simulink model "geometric_control__force_observer"  (R2021b)
settings: Solver=ode3  StartTime=0.0  StopTime=80  FixedStep=1e-2  RelTol=1e-3  EnableMultiTasking=on
libraries: sharedutil x7
settings Model: Creator=user
settings SolverCC: AlgebraicLoopSolver=TrustRegion  AutoInsertRateTranBlk=on
settings DataIOCC: LimitDataPoints=on  SaveFormat=Array  ReturnWorkspaceOutputs=off
settings OptimizationCC: ExpressionDepthLimit=2147483647  LifeSpan=inf
settings DebuggingCC: UnderspecifiedInitializationDetection=Classic  MergeDetectMultiDrivingBlocksExec=none  SolverPrmCheckMsg=warning  StateNameClashWarn=warning  SFUnexpectedBacktrackingDiag=warning  SFNoUnconditionalDefaultTransitionDiag=warning  SFExecutionAtInitializationDiag=none  SFMachineParentedDataDiag=warning  ArithmeticOperatorsInVariantConditions=warning
settings HardwareCC: ProdBitPerPointer=32  ProdBitPerSizeT=32  ProdBitPerPtrDiffT=32  ProdLargestAtomicFloat=None  ProdIntDivRoundTo=Undefined  ProdEndianess=Unspecified  ProdWordSize=32  ProdHWDeviceType=32-bit Generic
settings ModelReferenceCC: PropagateSignalLabelsOutOfModel=off
settings SFSimCC: SimUseLocalCustomCode=off  CustomCodeUndefinedFunction=UseInterfaceOnly
settings RTWCC: RTWUseLocalCustomCode=off
settings CodeAppCC: StateflowObjectComments=on
settings GRTTargetCC: TargetLangStandard=C89/C90 (ANSI)
settings ConfigComp: CovMetricSettings=dw  CovSaveCumulativeToWorkspaceVar=on  CovSaveSingleToWorkspaceVar=on  CovExternalEMLEnable=off

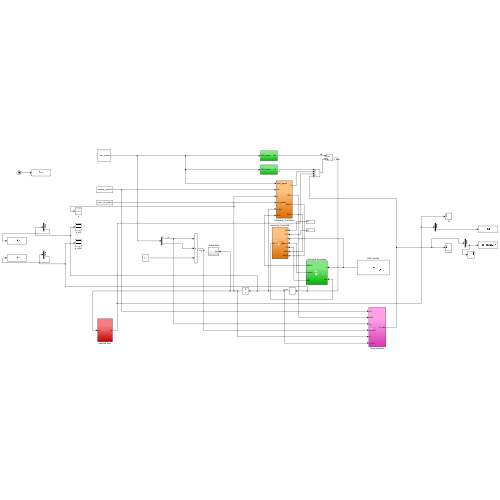
[thumbnail: Simulink's stored preview of the top-level diagram]
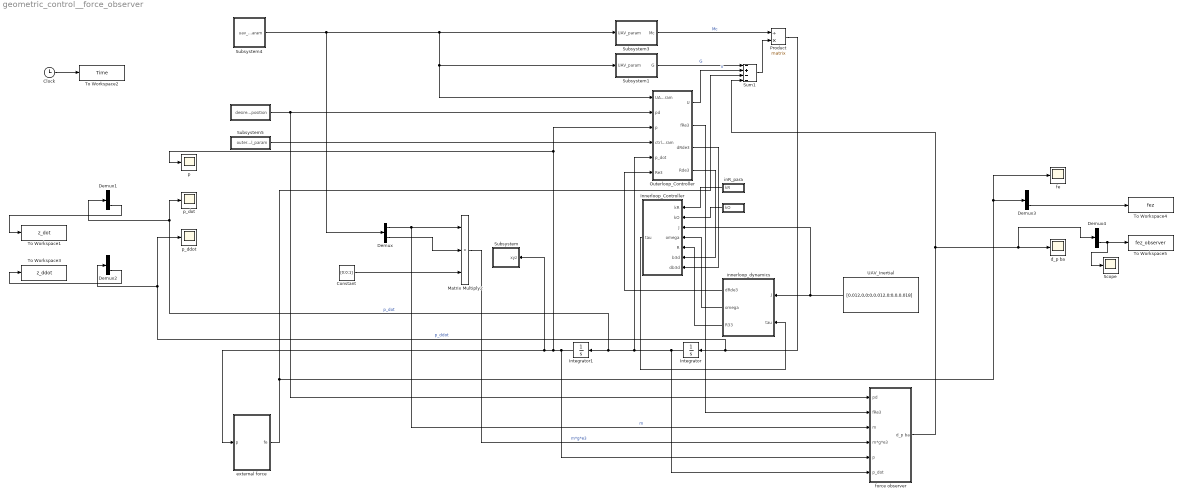
== system geometric_control__force_observer ==
  " " : Subsystem  mask{xd=3, yd=6, zd=10}
  "  " : Subsystem  mask{kO=diag([0.6,0.6,1])}
  "  Subsystem" : Subsystem
  Clock : Clock
  Constant : Constant  Value=[0;0;1]
  Demux : Demux  Outputs=2
  Demux{1..4} (4 alike) : Demux  Outputs=3
  Innerloop_Controller : Subsystem
  Integrator : Integrator  InitialCondition=[0;0;0]
  Integrator1 : Integrator  InitialCondition=[0;0;0]
  Matrix Multiply2 : Product  Inputs=3
  Outerloop_Controller : Subsystem
  Product : Product  Inputs=/*  Multiplication=Matrix(*)  RndMeth=Zero
  Scope : Scope
  Subsystem1 : Subsystem
  Subsystem3 : Subsystem
  Subsystem4 : Subsystem  mask{M=1.4, g=9.8}
  Subsystem5 : Subsystem  mask{kp1=0.1, kd1=1, kp2=0.5, kd2=3, kp3=0.05, kd3=0.5}
  Sum1 : Sum  Inputs=-+--
  To Workspace1 : ToWorkspace  VariableName=z_dot  SaveFormat=Structure With Time  SampleTime=-1
  To Workspace2 : ToWorkspace  VariableName=Time  SaveFormat=Timeseries  SampleTime=-1
  To Workspace3 : ToWorkspace  VariableName=z_ddot  SaveFormat=Structure With Time  SampleTime=-1
  To Workspace4 : ToWorkspace  VariableName=fez  SaveFormat=Structure With Time  SampleTime=-1
  To Workspace5 : ToWorkspace  VariableName=fez_observer  SaveFormat=Structure With Time  SampleTime=-1
  UAV_Inertial : Constant  Value=[0.012,0,0;0,0.012,0;0,0,0.018]
  d_p ba : Scope
  external force : Subsystem
  fe : Scope
  force observer : Subsystem
  inR_para : Subsystem  mask{kR=diag([5,5,4.7])}
  innerloop_dynamics : Subsystem
  p : Scope
  p_ddot : Scope
  p_dot : Scope
  wires:
  Subsystem3/1("Mc ") -> Product/1  "Mc"
  Product/1 -> p_ddot/1, Demux2/1, Integrator/1  "p_ddot"
  Subsystem4/1(uav_param) -> Outerloop_Controller/1(UAV_param), Subsystem1/1(UAV_param), Subsystem3/1(UAV_param), Demux/1
  Outerloop_Controller/1(U) -> Sum1/2  "u"
  Outerloop_Controller/3(dRde3) -> Innerloop_Controller/7(db3d)
  Outerloop_Controller/4(Rde3) -> Innerloop_Controller/6(b3d)
  UAV_Inertial/1 -> Innerloop_Controller/3(J), innerloop_dynamics/1(J)
  innerloop_dynamics/2(omega) -> Innerloop_Controller/4(omega)
  innerloop_dynamics/3(R33) -> Innerloop_Controller/5(R)
  Subsystem1/1("G ") -> Sum1/1  "G"
  Sum1/1 -> Product/2
  Innerloop_Controller/1(tau) -> innerloop_dynamics/2(tau)
  innerloop_dynamics/1(dRde3) -> Outerloop_Controller/6(Re3)
  Subsystem5/1(outer_ctrl_param) -> Outerloop_Controller/4(ctrl_param)
  Integrator/1 -> Demux1/1, p_dot/1, Integrator1/1, Outerloop_Controller/5(p_dot), force observer/6(p_dot)  "p_dot"
  "  "/1(kO) -> Innerloop_Controller/2(kO)
  inR_para/1(kR) -> Innerloop_Controller/1(kR)
  Demux/1 -> force observer/3(m), Matrix Multiply2/1  "m"
  Demux/2 -> Matrix Multiply2/2
  Constant/1 -> Matrix Multiply2/3
  " "/1(desired_position) -> Outerloop_Controller/2(pd), force observer/1(pd)
  Integrator1/1 -> external force/1(p), "  Subsystem"/1(xyz), Outerloop_Controller/3(p), p/1, force observer/5(p)
  external force/1(fe) -> Demux3/1, fe/1, Sum1/3
  Outerloop_Controller/2(fRe3) -> force observer/2(fRe3)
  Matrix Multiply2/1 -> force observer/4(m*g*e3)  "m*g*e3"
  force observer/1(d_p ba) -> Sum1/4, Demux4/1, d_p ba/1
  Clock/1 -> To Workspace2/1
  Demux1/3 -> To Workspace1/1
  Demux2/3 -> To Workspace3/1
  Demux3/3 -> To Workspace4/1
  Demux4/3 -> Scope/1, To Workspace5/1

== system geometric_control__force_observer/  ==
  Constant : Constant  Value=xd
  Constant1 : Constant  Value=zd
  Constant2 : Constant  Value=yd
  Mux : Mux  Inputs=3
  desired_position : Outport
  wires:
  Constant/1 -> Mux/1
  Constant2/1 -> Mux/2
  Mux/1 -> desired_position/1
  Constant1/1 -> Mux/3

== system geometric_control__force_observer/   ==
  Constant1 : Constant  Value=kO
  kO : Outport
  wires:
  Constant1/1 -> kO/1

== system geometric_control__force_observer/  Subsystem ==
  xyz : Inport
  Demux : Demux  Outputs=3
  To Workspace : ToWorkspace  VariableName=x  SaveFormat=Structure With Time  SampleTime=-1
      settings: Save2DSignal=2-D array (concatenate along first dimension)
  To Workspace2 : ToWorkspace  VariableName=y  SaveFormat=Structure With Time  SampleTime=-1
      settings: Save2DSignal=2-D array (concatenate along first dimension)
  To Workspace3 : ToWorkspace  VariableName=z  SaveFormat=Structure With Time  SampleTime=-1
      settings: Save2DSignal=2-D array (concatenate along first dimension)
  wires:
  Demux/3 -> To Workspace3/1
  Demux/1 -> To Workspace/1
  Demux/2 -> To Workspace2/1
  xyz/1 -> Demux/1

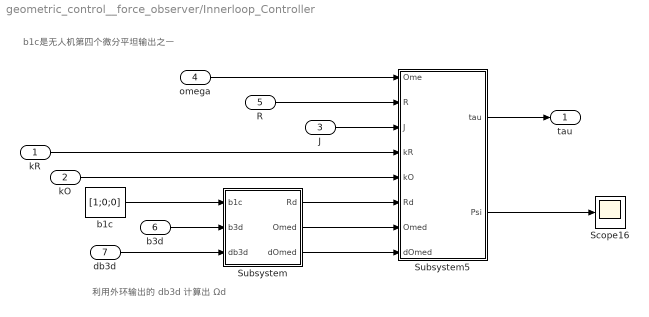
== system geometric_control__force_observer/Innerloop_Controller ==
  note: 利用外环输出的 db3d 计算出 Ωd
  note: b1c是无人机第四个微分平坦输出之一
  kR : Inport
  kO : Inport  Port=2
  J : Inport  Port=3
  omega : Inport  Port=4
  R : Inport  Port=5
  b3d : Inport  Port=6
  db3d : Inport  Port=7
  Scope16 : Scope
  Subsystem : Subsystem
  Subsystem5 : Subsystem
  b1c : Constant  Value=[1;0;0]
  tau : Outport
  wires:
  b1c/1 -> Subsystem/1(b1c)
  Subsystem5/2(Psi) -> Scope16/1
  db3d/1 -> Subsystem/3(db3d)
  kR/1 -> Subsystem5/4(kR)
  Subsystem/2(Omed) -> Subsystem5/7(Omed)
  Subsystem/1(Rd) -> Subsystem5/6(Rd)
  b3d/1 -> Subsystem/2(b3d)
  Subsystem/3(dOmed) -> Subsystem5/8(dOmed)
  kO/1 -> Subsystem5/5(kO)
  omega/1 -> Subsystem5/1(Ome)
  R/1 -> Subsystem5/2(R)
  J/1 -> Subsystem5/3(J)
  Subsystem5/1(tau) -> tau/1

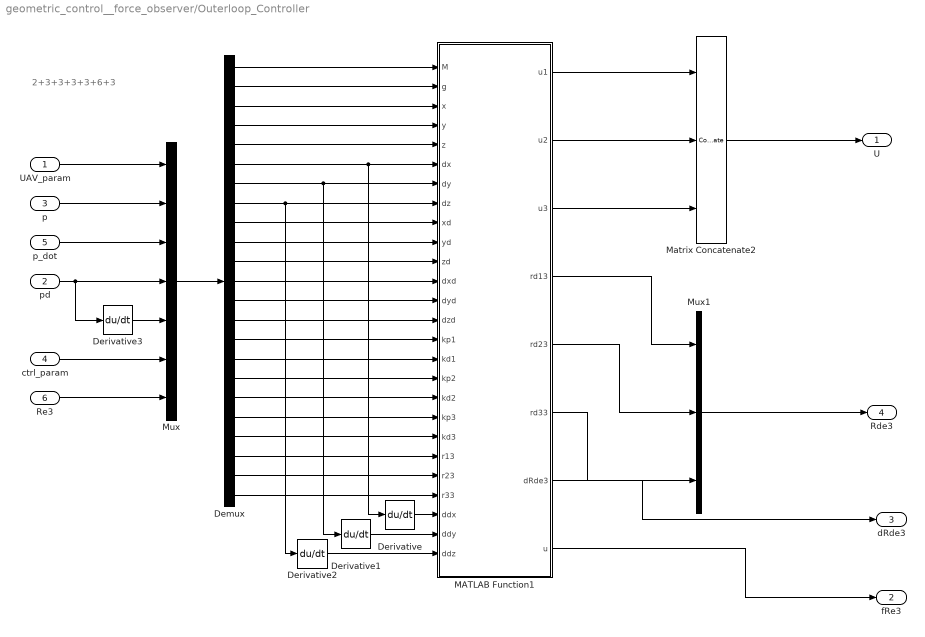
== system geometric_control__force_observer/Outerloop_Controller ==
  note: 2+3+3+3+3+6+3
  UAV_param : Inport
  pd : Inport  Port=2
  p : Inport  Port=3
  ctrl_param : Inport  Port=4
  p_dot : Inport  Port=5
  Re3 : Inport  Port=6
  Demux : Demux  Outputs=23
  Derivative{,1..3} (4 alike) : Derivative
  MATLAB Function1 : MATLAB Function  TreatAsAtomicUnit=on
  Matrix Concatenate2 : Concatenate  NumInputs=3  Mode=Multidimensional array
  Mux : Mux  Inputs=7
  Mux1 : Mux  Inputs=3
  U : Outport
  fRe3 : Outport  Port=2
  dRde3 : Outport  Port=3
  Rde3 : Outport  Port=4
  wires:
  Matrix Concatenate2/1 -> U/1
  UAV_param/1 -> Mux/1
  Mux/1 -> Demux/1
  Mux1/1 -> Rde3/1
  p_dot/1 -> Mux/3
  ctrl_param/1 -> Mux/6
  Re3/1 -> Mux/7
  p/1 -> Mux/2
  Demux/1 -> MATLAB Function1/1(M)
  Demux/2 -> MATLAB Function1/2(g)
  Demux/3 -> MATLAB Function1/3(x)
  Demux/4 -> MATLAB Function1/4(y)
  Demux/5 -> MATLAB Function1/5(z)
  Demux/6 -> Derivative/1, MATLAB Function1/6(dx)
  Demux/7 -> MATLAB Function1/7(dy), Derivative1/1
  Demux/8 -> Derivative2/1, MATLAB Function1/8(dz)
  Demux/9 -> MATLAB Function1/9(xd)
  Demux/10 -> MATLAB Function1/10(yd)
  Demux/11 -> MATLAB Function1/11(zd)
  Demux/12 -> MATLAB Function1/12(dxd)
  Demux/13 -> MATLAB Function1/13(dyd)
  Demux/14 -> MATLAB Function1/14(dzd)
  Demux/15 -> MATLAB Function1/15(kp1)
  Demux/16 -> MATLAB Function1/16(kd1)
  Demux/17 -> MATLAB Function1/17(kp2)
  Demux/18 -> MATLAB Function1/18(kd2)
  Demux/19 -> MATLAB Function1/19(kp3)
  Demux/20 -> MATLAB Function1/20(kd3)
  Demux/21 -> MATLAB Function1/21(r13)
  Demux/22 -> MATLAB Function1/22(r23)
  Demux/23 -> MATLAB Function1/23(r33)
  MATLAB Function1/1(u1) -> Matrix Concatenate2/1
  MATLAB Function1/2(u2) -> Matrix Concatenate2/2
  MATLAB Function1/3(u3) -> Matrix Concatenate2/3
  MATLAB Function1/4(rd13) -> Mux1/1
  MATLAB Function1/5(rd23) -> Mux1/2
  MATLAB Function1/6(rd33) -> Mux1/3
  MATLAB Function1/7(dRde3) -> dRde3/1
  Derivative/1 -> MATLAB Function1/24(ddx)
  Derivative1/1 -> MATLAB Function1/25(ddy)
  Derivative2/1 -> MATLAB Function1/26(ddz)
  pd/1 -> Derivative3/1, Mux/4
  Derivative3/1 -> Mux/5
  MATLAB Function1/8(u) -> fRe3/1

== system geometric_control__force_observer/Subsystem1 ==
  UAV_param : Inport
  G1 : Fcn  Expr=0*u(1)
  G2 : Fcn  Expr=0*u(1)
  G3 : Fcn  Expr=u(1)*u(2)
  Matrix Concatenate2 : Concatenate  NumInputs=3  Mode=Multidimensional array
  "G " : Outport
  wires:
  UAV_param/1 -> G1/1, G2/1, G3/1
  Matrix Concatenate2/1 -> "G "/1
  G3/1 -> Matrix Concatenate2/3
  G2/1 -> Matrix Concatenate2/2
  G1/1 -> Matrix Concatenate2/1

== system geometric_control__force_observer/Subsystem3 ==
  UAV_param : Inport
  Matrix Concatenate2 : Concatenate  NumInputs=3  Mode=Multidimensional array  ConcatenateDimension=2
  Subsystem : Subsystem
  Subsystem1 : Subsystem
  Subsystem2 : Subsystem
  "Mc " : Outport
  wires:
  UAV_param/1 -> Subsystem/1((S,p)), Subsystem1/1((S,p)), Subsystem2/1((S,p))
  Matrix Concatenate2/1 -> "Mc "/1
  Subsystem2/1(Mc3) -> Matrix Concatenate2/3
  Subsystem1/1(Mc2) -> Matrix Concatenate2/2
  Subsystem/1(Mc1) -> Matrix Concatenate2/1

== system geometric_control__force_observer/Subsystem4 ==
  Constant : Constant  Value=M
  Constant2 : Constant  Value=g
  Mux : Mux  Inputs=2
  uav_param : Outport
  wires:
  Constant/1 -> Mux/1
  Constant2/1 -> Mux/2
  Mux/1 -> uav_param/1

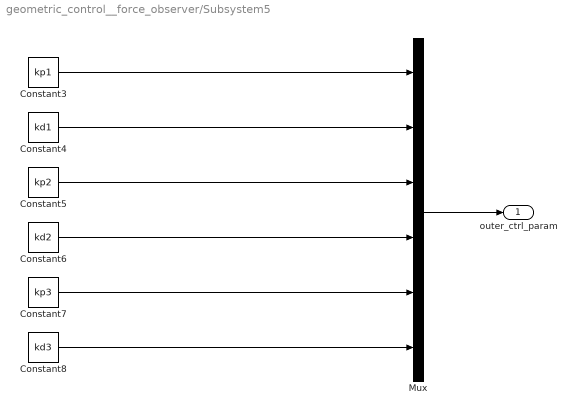
== system geometric_control__force_observer/Subsystem5 ==
  Constant3 : Constant  Value=kp1
  Constant4 : Constant  Value=kd1
  Constant5 : Constant  Value=kp2
  Constant6 : Constant  Value=kd2
  Constant7 : Constant  Value=kp3
  Constant8 : Constant  Value=kd3
  Mux : Mux  Inputs=6
  outer_ctrl_param : Outport
  wires:
  Mux/1 -> outer_ctrl_param/1
  Constant3/1 -> Mux/1
  Constant4/1 -> Mux/2
  Constant5/1 -> Mux/3
  Constant6/1 -> Mux/4
  Constant7/1 -> Mux/5
  Constant8/1 -> Mux/6

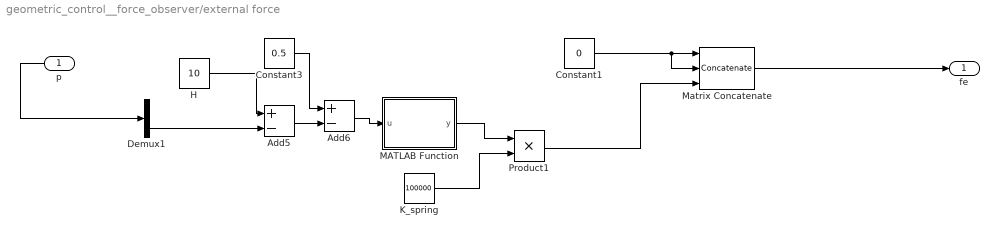
== system geometric_control__force_observer/external force ==
  p : Inport
  Add5 : Sum  Inputs=+-
  Add6 : Sum  Inputs=+-
  Constant1 : Constant  Value=0
  Constant3 : Constant  Value=0.5
  Demux1 : Demux  Outputs=3
  H : Constant  Value=10
  K_spring : Constant  Value=100000
  MATLAB Function : MATLAB Function  TreatAsAtomicUnit=on
  Matrix Concatenate : Concatenate  NumInputs=3  Mode=Multidimensional array
  Product1 : Product
  fe : Outport
  wires:
  H/1 -> Add5/1
  Product1/1 -> Matrix Concatenate/3
  Add5/1 -> Add6/2
  Matrix Concatenate/1 -> fe/1
  MATLAB Function/1(y) -> Product1/1
  K_spring/1 -> Product1/2
  Add6/1 -> MATLAB Function/1(u)
  p/1 -> Demux1/1
  Demux1/3 -> Add5/2
  Constant3/1 -> Add6/1
  Constant1/1 -> Matrix Concatenate/2, Matrix Concatenate/1

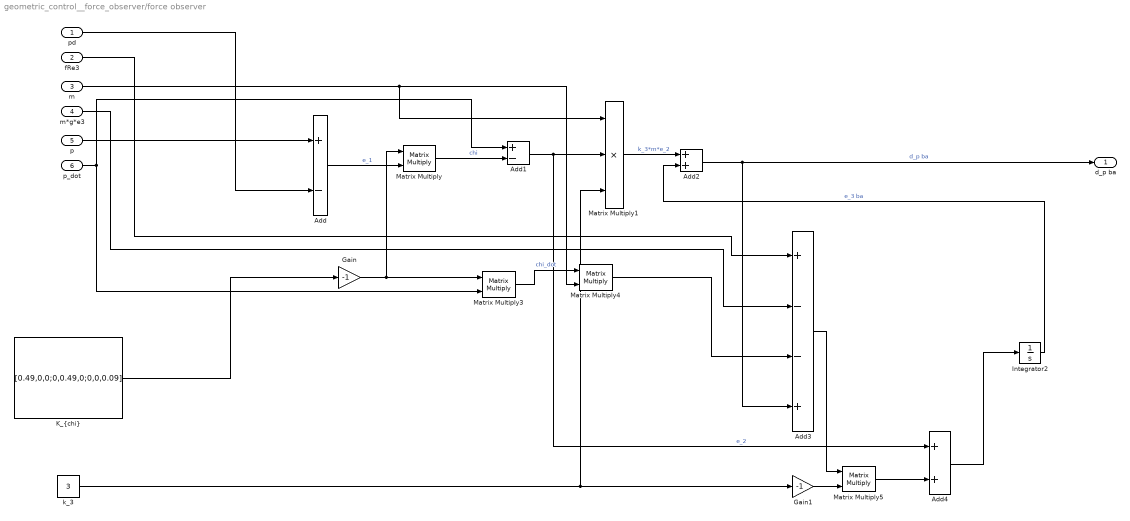
== system geometric_control__force_observer/force observer ==
  pd : Inport
  fRe3 : Inport  Port=2
  m : Inport  Port=3
  m*g*e3 : Inport  Port=4
  p : Inport  Port=5
  p_dot : Inport  Port=6
  Add : Sum  Inputs=+-
  Add1 : Sum  Inputs=+-
  Add2 : Sum
  Add3 : Sum  Inputs=+--+
  Add4 : Sum
  Gain : Gain  Gain=-1
  Gain1 : Gain  Gain=-1
  Integrator2 : Integrator
  "K_{chi}" : Constant  Value=[0.49,0,0;0,0.49,0;0,0,0.09]
  Matrix Multiply{,3..5} (4 alike) : Product  Multiplication=Matrix(*)
  Matrix Multiply1 : Product  Inputs=3
  k_3 : Constant  Value=3
  d_p ba : Outport
  wires:
  Add2/1 -> d_p ba/1, Add3/4  "d_p ba"
  Gain/1 -> Matrix Multiply/1, Matrix Multiply3/1
  Add4/1 -> Integrator2/1
  p_dot/1 -> Add1/1, Matrix Multiply3/2
  p/1 -> Add/1
  Matrix Multiply4/1 -> Add3/3
  Add1/1 -> Add4/1, Matrix Multiply1/2  "e_2"
  k_3/1 -> Matrix Multiply1/3, Gain1/1
  Add/1 -> Matrix Multiply/2  "e_1"
  Matrix Multiply1/1 -> Add2/1  "k_3*m*e_2"
  fRe3/1 -> Add3/1
  Integrator2/1 -> Add2/2  "e_3 ba"
  m/1 -> Matrix Multiply1/1, Matrix Multiply4/2
  Matrix Multiply3/1 -> Matrix Multiply4/1  "chi_dot"
  Matrix Multiply/1 -> Add1/2  "chi"
  "K_{chi}"/1 -> Gain/1
  Matrix Multiply5/1 -> Add4/2
  Add3/1 -> Matrix Multiply5/1
  Gain1/1 -> Matrix Multiply5/2
  m*g*e3/1 -> Add3/2
  pd/1 -> Add/2

== system geometric_control__force_observer/inR_para ==
  Constant : Constant  Value=kR
  kR : Outport
  wires:
  Constant/1 -> kR/1

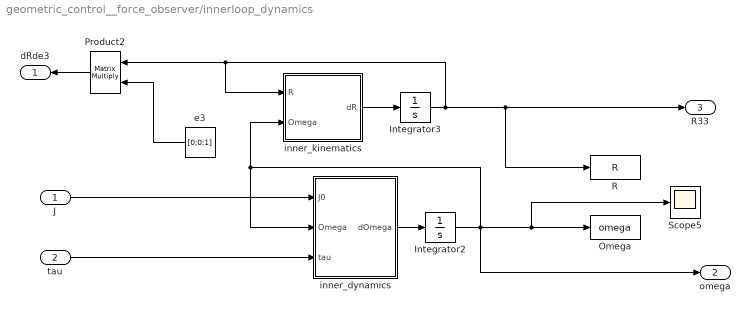
== system geometric_control__force_observer/innerloop_dynamics ==
  J : Inport
  tau : Inport  Port=2
  Integrator2 : Integrator  InitialCondition=[0;0;0]
  Integrator3 : Integrator  InitialCondition=[1,0,0;0,1,0;0,0,1]
  Omega : ToWorkspace  VariableName=omega  SampleTime=-1
  Product2 : Product  Multiplication=Matrix(*)  RndMeth=Zero
  R : ToWorkspace  VariableName=R  SampleTime=-1
  Scope5 : Scope
  e3 : Constant  Value=[0;0;1]
  inner_dynamics : Subsystem
  inner_kinematics : Subsystem
  dRde3 : Outport
  omega : Outport  Port=2
  R33 : Outport  Port=3
  wires:
  inner_kinematics/1(dR) -> Integrator3/1
  Product2/1 -> dRde3/1
  Integrator3/1 -> inner_kinematics/1(R), Product2/1, R/1, R33/1
  Integrator2/1 -> Omega/1, Scope5/1, inner_dynamics/2(Omega), inner_kinematics/2(Omega), omega/1
  e3/1 -> Product2/2
  inner_dynamics/1(dOmega) -> Integrator2/1
  J/1 -> inner_dynamics/1(J0)
  tau/1 -> inner_dynamics/3(tau)

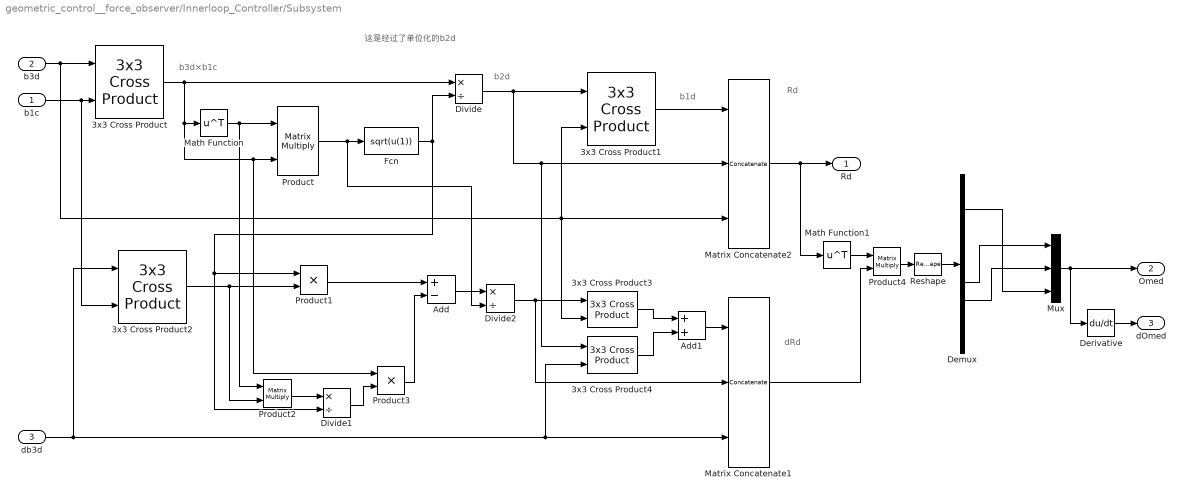
== system geometric_control__force_observer/Innerloop_Controller/Subsystem ==
  note: 这是经过了单位化的b2d
  note: b3d×b1c
  note: dRd
  note: Rd
  note: b1d
  note: b2d
  b1c : Inport
  b3d : Inport  Port=2
  db3d : Inport  Port=3
  3x3 Cross Product{,1..4} (5 alike) : sharedutil/3x3 Cross Product  aMode=aMode
      settings: SourceProductBaseCode=AE,PW,DR,MT,UV,VE
  Add : Sum  Inputs=+-
  Add1 : Sum
  Demux : Demux  Outputs=9
  Derivative : Derivative
  Divide : Product  Inputs=*/
  Divide1 : Product  Inputs=*/
  Divide2 : Product  Inputs=*/
  Fcn : Fcn  Expr=sqrt(u(1))
  Math Function : Math  Operator=transpose  SignedPower=on  SaturateOnIntegerOverflow=on
  Math Function1 : Math  Operator=transpose  SignedPower=on  SaturateOnIntegerOverflow=on
  Matrix Concatenate1 : Concatenate  NumInputs=3  Mode=Multidimensional array  ConcatenateDimension=2
  Matrix Concatenate2 : Concatenate  NumInputs=3  Mode=Multidimensional array  ConcatenateDimension=2
  Mux : Mux  Inputs=3
  Product : Product  Multiplication=Matrix(*)  RndMeth=Zero
  Product1 : Product  RndMeth=Zero
  Product2 : Product  Multiplication=Matrix(*)  RndMeth=Zero
  Product3 : Product  RndMeth=Zero
  Product4 : Product  Multiplication=Matrix(*)  RndMeth=Zero
  Reshape : Reshape
  Rd : Outport
  Omed : Outport  Port=2
  dOmed : Outport  Port=3
  wires:
  b3d/1 -> 3x3 Cross Product1/2, Matrix Concatenate2/3, 3x3 Cross Product3/2, 3x3 Cross Product/1
  b1c/1 -> 3x3 Cross Product2/2, 3x3 Cross Product/2
  3x3 Cross Product/1 -> Product3/1, Product/2, Math Function/1, Divide/1
  Math Function/1 -> Product/1, Product2/1
  Product/1 -> Divide2/2, Fcn/1
  Fcn/1 -> Divide1/2, Product1/1, Divide/2
  3x3 Cross Product1/1 -> Matrix Concatenate2/1
  db3d/1 -> 3x3 Cross Product2/1, 3x3 Cross Product4/2, Matrix Concatenate1/3
  3x3 Cross Product2/1 -> Product2/2, Product1/2
  Product1/1 -> Add/1
  Product2/1 -> Divide1/1
  Divide1/1 -> Product3/2
  Product3/1 -> Add/2
  Add/1 -> Divide2/1
  Divide2/1 -> 3x3 Cross Product3/1, Matrix Concatenate1/2
  3x3 Cross Product3/1 -> Add1/1
  3x3 Cross Product4/1 -> Add1/2
  Add1/1 -> Matrix Concatenate1/1
  Divide/1 -> 3x3 Cross Product4/1, Matrix Concatenate2/2, 3x3 Cross Product1/1
  Matrix Concatenate2/1 -> Math Function1/1, Rd/1
  Matrix Concatenate1/1 -> Product4/2
  Math Function1/1 -> Product4/1
  Demux/2 -> Mux/3
  Demux/6 -> Mux/1
  Demux/7 -> Mux/2
  Mux/1 -> Derivative/1, Omed/1
  Derivative/1 -> dOmed/1
  Reshape/1 -> Demux/1
  Product4/1 -> Reshape/1

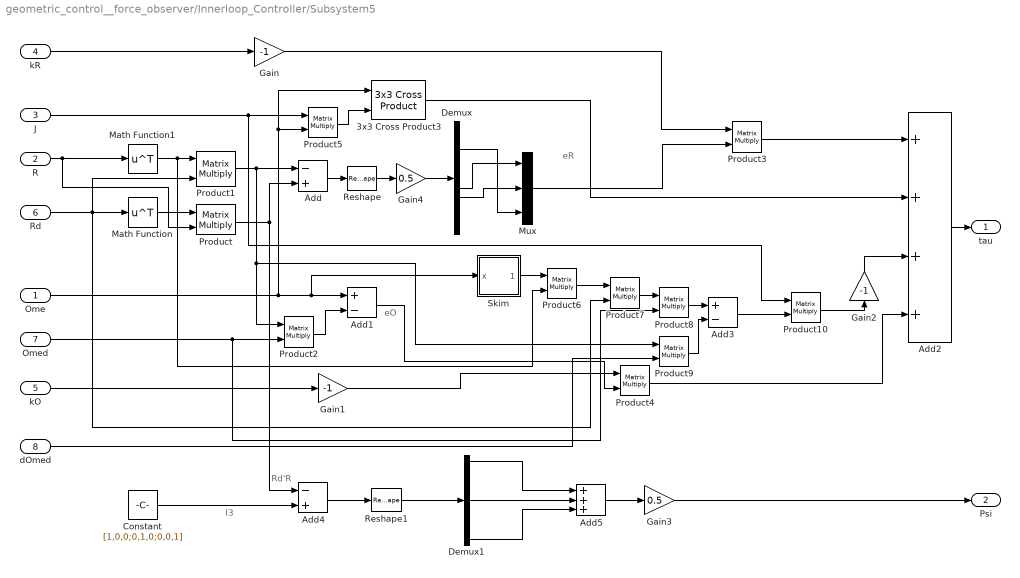
== system geometric_control__force_observer/Innerloop_Controller/Subsystem5 ==
  note: Rd'R
  note: I3
  note: eO
  note: eR
  Ome : Inport
  R : Inport  Port=2
  J : Inport  Port=3
  kR : Inport  Port=4
  kO : Inport  Port=5
  Rd : Inport  Port=6
  Omed : Inport  Port=7
  dOmed : Inport  Port=8
  3x3 Cross Product3 : sharedutil/3x3 Cross Product  aMode=aMode
      settings: SourceProductBaseCode=AE,PW,DR,MT,UV,VE
  Add : Sum  Inputs=-+
  Add1 : Sum  Inputs=+-
  Add2 : Sum  Inputs=++++
  Add3 : Sum  Inputs=+-
  Add4 : Sum  Inputs=-+
  Add5 : Sum  Inputs=+++
  Constant : Constant  Value=[1,0,0;0,1,0;0,0,1]
  Demux : Demux  Outputs=9
  Demux1 : Demux  Outputs=9
  Gain : Gain  Gain=-1
  Gain1 : Gain  Gain=-1
  Gain2 : Gain  Gain=-1
  Gain3 : Gain  Gain=0.5
  Gain4 : Gain  Gain=0.5
  Math Function : Math  Operator=transpose  SignedPower=on  SaturateOnIntegerOverflow=on
  Math Function1 : Math  Operator=transpose  SignedPower=on  SaturateOnIntegerOverflow=on
  Mux : Mux  Inputs=3
  Product{,1..10} (11 alike) : Product  Multiplication=Matrix(*)  RndMeth=Zero
  Reshape : Reshape
  Reshape1 : Reshape
  Skim : Subsystem
  tau : Outport
  Psi : Outport  Port=2
  wires:
  R/1 -> Product/2, Math Function1/1
  Rd/1 -> Product1/2, Math Function/1, Product7/2
  Math Function1/1 -> Product6/2, Product1/1
  Product1/1 -> Product9/1, Product2/1, Add/1
  Product/1 -> Add/2, Add4/1
  Add/1 -> Reshape/1
  Reshape/1 -> Gain4/1
  Demux/2 -> Mux/3
  Demux/6 -> Mux/1
  Demux/7 -> Mux/2
  Omed/1 -> Product8/2, Product2/2
  Ome/1 -> 3x3 Cross Product3/1, Product5/2, Skim/1(x), Add1/1
  Product2/1 -> Add1/2
  kR/1 -> Gain/1
  Mux/1 -> Product3/2
  Gain/1 -> Product3/1
  kO/1 -> Gain1/1
  Gain1/1 -> Product4/1
  Add1/1 -> Product4/2
  Add2/1 -> tau/1
  J/1 -> Product10/1, Product5/1
  Product5/1 -> 3x3 Cross Product3/2
  3x3 Cross Product3/1 -> Add2/2
  Product3/1 -> Add2/1
  Product4/1 -> Add2/4
  Skim/1(sk(x)) -> Product6/1
  Product6/1 -> Product7/1
  Product7/1 -> Product8/1
  Product8/1 -> Add3/1
  dOmed/1 -> Product9/2
  Product9/1 -> Add3/2
  Add3/1 -> Product10/2
  Product10/1 -> Gain2/1
  Gain2/1 -> Add2/3
  Math Function/1 -> Product/1
  Constant/1 -> Add4/2
  Reshape1/1 -> Demux1/1
  Add4/1 -> Reshape1/1
  Demux1/1 -> Add5/1
  Demux1/5 -> Add5/2
  Demux1/9 -> Add5/3
  Add5/1 -> Gain3/1
  Gain3/1 -> Psi/1
  Gain4/1 -> Demux/1

== system geometric_control__force_observer/Subsystem3/Subsystem ==
  (S,p) : Inport
  Matrix Concatenate2 : Concatenate  NumInputs=3  Mode=Multidimensional array
  Mc11 : Fcn  Expr=u(1)
  Mc21 : Fcn  Expr=0*u(1)
  Mc31 : Fcn  Expr=0*u(1)
  Mc1 : Outport
  wires:
  (S,p)/1 -> Mc11/1, Mc31/1, Mc21/1
  Mc11/1 -> Matrix Concatenate2/1
  Mc21/1 -> Matrix Concatenate2/2
  Mc31/1 -> Matrix Concatenate2/3
  Matrix Concatenate2/1 -> Mc1/1

== system geometric_control__force_observer/Subsystem3/Subsystem1 ==
  (S,p) : Inport
  Matrix Concatenate2 : Concatenate  NumInputs=3  Mode=Multidimensional array
  Mc12 : Fcn  Expr=0*u(1)
  Mc22 : Fcn  Expr=u(1)
  Mc32 : Fcn  Expr=0*u(1)
  Mc2 : Outport
  wires:
  (S,p)/1 -> Mc22/1, Mc32/1, Mc12/1
  Mc12/1 -> Matrix Concatenate2/1
  Mc22/1 -> Matrix Concatenate2/2
  Mc32/1 -> Matrix Concatenate2/3
  Matrix Concatenate2/1 -> Mc2/1

== system geometric_control__force_observer/Subsystem3/Subsystem2 ==
  (S,p) : Inport
  Matrix Concatenate2 : Concatenate  NumInputs=3  Mode=Multidimensional array
  Mc13 : Fcn  Expr=0*u(1)
  Mc23 : Fcn  Expr=0*u(1)
  Mc33 : Fcn  Expr=u(1)
  Mc3 : Outport
  wires:
  (S,p)/1 -> Mc23/1, Mc33/1, Mc13/1
  Mc13/1 -> Matrix Concatenate2/1
  Mc23/1 -> Matrix Concatenate2/2
  Mc33/1 -> Matrix Concatenate2/3
  Matrix Concatenate2/1 -> Mc3/1

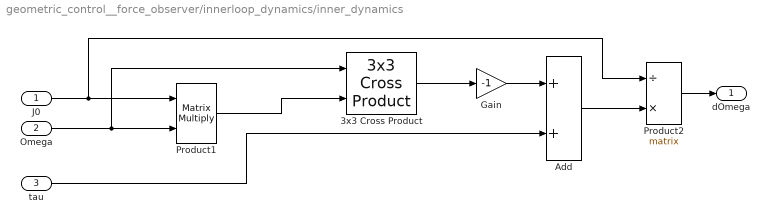
== system geometric_control__force_observer/innerloop_dynamics/inner_dynamics ==
  J0 : Inport
  Omega : Inport  Port=2
  tau : Inport  Port=3
  3x3 Cross Product : sharedutil/3x3 Cross Product  aMode=aMode
      settings: SourceProductBaseCode=AE,PW,DR,MT,UV,VE
  Add : Sum
  Gain : Gain  Gain=-1
  Product1 : Product  Multiplication=Matrix(*)  RndMeth=Zero
  Product2 : Product  Inputs=/*  Multiplication=Matrix(*)  RndMeth=Zero
  dOmega : Outport
  wires:
  J0/1 -> Product1/1, Product2/1
  Omega/1 -> 3x3 Cross Product/1, Product1/2
  Product1/1 -> 3x3 Cross Product/2
  3x3 Cross Product/1 -> Gain/1
  Gain/1 -> Add/1
  tau/1 -> Add/2
  Add/1 -> Product2/2
  Product2/1 -> dOmega/1

== system geometric_control__force_observer/innerloop_dynamics/inner_kinematics ==
  R : Inport
  Omega : Inport  Port=2
  Product1 : Product  Multiplication=Matrix(*)  RndMeth=Zero
  Skew : Subsystem
  dR : Outport
  wires:
  Omega/1 -> Skew/1(Omega)
  R/1 -> Product1/1
  Skew/1(OmegaX) -> Product1/2
  Product1/1 -> dR/1

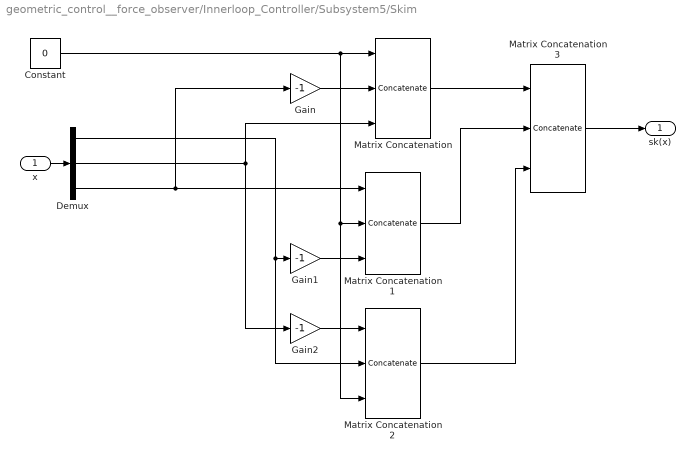
== system geometric_control__force_observer/Innerloop_Controller/Subsystem5/Skim ==
  x : Inport
  Constant : Constant  Value=0
  Demux : Demux  Outputs=3
  Gain : Gain  Gain=-1
  Gain1 : Gain  Gain=-1
  Gain2 : Gain  Gain=-1
  Matrix Concatenation : Concatenate  NumInputs=3  Mode=Multidimensional array  ConcatenateDimension=2
  Matrix Concatenation1 : Concatenate  NumInputs=3  Mode=Multidimensional array  ConcatenateDimension=2
  Matrix Concatenation2 : Concatenate  NumInputs=3  Mode=Multidimensional array  ConcatenateDimension=2
  Matrix Concatenation3 : Concatenate  NumInputs=3  Mode=Multidimensional array
  sk(x) : Outport
  wires:
  x/1 -> Demux/1
  Matrix Concatenation/1 -> Matrix Concatenation3/1
  Matrix Concatenation1/1 -> Matrix Concatenation3/2
  Matrix Concatenation2/1 -> Matrix Concatenation3/3
  Matrix Concatenation3/1 -> sk(x)/1
  Gain/1 -> Matrix Concatenation/2
  Gain1/1 -> Matrix Concatenation1/3
  Gain2/1 -> Matrix Concatenation2/1
  Constant/1 -> Matrix Concatenation/1, Matrix Concatenation1/2, Matrix Concatenation2/3
  Demux/3 -> Gain/1, Matrix Concatenation1/1
  Demux/2 -> Matrix Concatenation/3, Gain2/1
  Demux/1 -> Gain1/1, Matrix Concatenation2/2

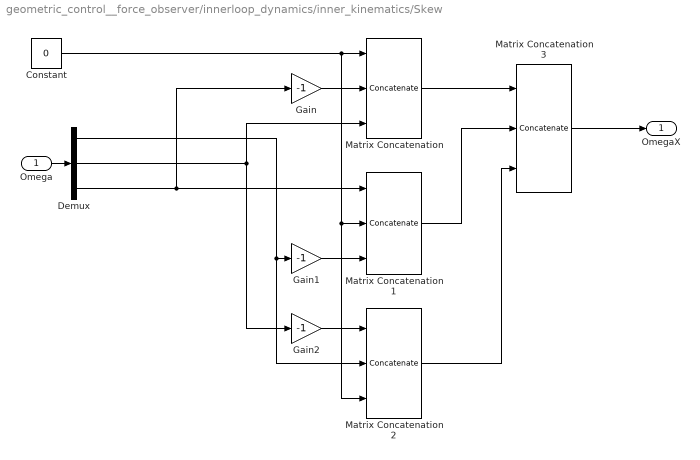
== system geometric_control__force_observer/innerloop_dynamics/inner_kinematics/Skew ==
  Omega : Inport
  Constant : Constant  Value=0
  Demux : Demux  Outputs=3
  Gain : Gain  Gain=-1
  Gain1 : Gain  Gain=-1
  Gain2 : Gain  Gain=-1
  Matrix Concatenation : Concatenate  NumInputs=3  Mode=Multidimensional array  ConcatenateDimension=2
  Matrix Concatenation1 : Concatenate  NumInputs=3  Mode=Multidimensional array  ConcatenateDimension=2
  Matrix Concatenation2 : Concatenate  NumInputs=3  Mode=Multidimensional array  ConcatenateDimension=2
  Matrix Concatenation3 : Concatenate  NumInputs=3  Mode=Multidimensional array
  OmegaX : Outport
  wires:
  Omega/1 -> Demux/1
  Matrix Concatenation/1 -> Matrix Concatenation3/1
  Matrix Concatenation1/1 -> Matrix Concatenation3/2
  Matrix Concatenation2/1 -> Matrix Concatenation3/3
  Matrix Concatenation3/1 -> OmegaX/1
  Gain/1 -> Matrix Concatenation/2
  Gain1/1 -> Matrix Concatenation1/3
  Gain2/1 -> Matrix Concatenation2/1
  Constant/1 -> Matrix Concatenation/1, Matrix Concatenation1/2, Matrix Concatenation2/3
  Demux/3 -> Gain/1, Matrix Concatenation1/1
  Demux/2 -> Matrix Concatenation/3, Gain2/1
  Demux/1 -> Gain1/1, Matrix Concatenation2/2

== matlab function geometric_control__force_observer/external force/MATLAB Function ==
  data: u input; y output
function y = fcn(u)

if (u>0)&&(u<=0.5)
    y=u;
elseif (u>0.5)
        y=50;
else
    y=0;
end

== matlab function geometric_control__force_observer/Outerloop_Controller/MATLAB Function1 ==
  data: M input; g input; x input; y input; z input; dx input; dy input; dz input; u1 output; u2 output; u3 output; xd input; yd input; zd input; dxd input; dyd input; dzd input; kp1 input; kd1 input; kp2 input; kd2 input; kp3 input; kd3 input; r13 input; r23 input; r33 input; rd13 output; rd23 output; rd33 output; dRde3 output; ddx input; ddy input; ddz input; u output
function [u1,u2,u3,rd13,rd23,rd33,dRde3,u] = fcn(M,g,x,y,z,dx,dy,dz,xd,yd,zd,dxd,dyd,dzd,kp1,kd1,kp2,kd2,kp3,kd3,r13,r23,r33,ddx,ddy,ddz)
e3=[0;0;1];
Re3=[r13;r23;r33];

texi=[x-xd;y-yd;z-zd];
dtexi=[dx-dxd;dy-dyd;dz-dzd];
tdexi=[dx-dxd;dy-dyd;dz-dzd];
dtdexi=[ddx;ddy;ddz];

kpxi=diag([kp1,kp2,kp3]);
kdxi=diag([kd1,kd2,kd3]);

A  = -kpxi*texi-kdxi*tdexi+M*g*e3;
dA = -kpxi*dtexi-kdxi*dtdexi;
MA = sqrt(A'*A);
Rde3 = A/MA;
f = A'*(Re3);
u = f*(Re3);
%% 外环输出
u1 = u(1);
u2 = u(2);
u3 = u(3);

rd13=Rde3(1);
rd23=Rde3(2);
rd33=Rde3(3);

dTRde3=1/MA*(eye(3)-A*A'/(MA)^2)*dA;

dRde3=1/f*(eye(3)-Rde3*(Re3)')*dTRde3;
